simulink model "simulink_controller"  (R2021a)
settings: Solver=FixedStepAuto  StartTime=0.0  StopTime=10.0  RelTol=1e-3
model workspace (MAT data in the model file):
  SL_ROS_VariableLengthArrays_MaxSizes.CommonInfo.ArrayTruncateAction = 'EmitWarning'
  SL_ROS_VariableLengthArrays_MaxSizes.MsgTypeMap = containers.Map
  SL_ROS_VariableLengthArrays_MaxSizes.MsgTypeMap.serialization.keys = {'std_msgs/Float64MultiArray'}
  SL_ROS_VariableLengthArrays_MaxSizes.MsgTypeMap.serialization.values{1}.PropertyName = 'data'
  SL_ROS_VariableLengthArrays_MaxSizes.MsgTypeMap.serialization.values{1}.DataType = 'double'
  SL_ROS_VariableLengthArrays_MaxSizes.MsgTypeMap.serialization.values{1}.MaxLength = 6
  SL_ROS_VariableLengthArrays_MaxSizes.MsgTypeMap.serialization.uniformity = 0
  SL_ROS_VariableLengthArrays_MaxSizes.MsgTypeMap.serialization.keyType = 'char'
  SL_ROS_VariableLengthArrays_MaxSizes.MsgTypeMap.serialization.valueType = 'any'
libraries: ros2lib x3
settings Model: Creator=legacy  LastModifiedBy=legacy
settings OptimizationCC: EnhancedBackFolding=on  PassReuseOutputArgsThreshold=0  ZeroExternalMemoryAtStartup=off  ZeroInternalMemoryAtStartup=off  MaxStackSize=64  OptimizeBlockOrder=speed  DifferentSizesBufferReuse=on  OptimizationCustomize=off
settings DebuggingCC: ParameterTunabilityLossMsg=error
settings HardwareCC: ProdBitPerLong=64  ProdHWDeviceType=Intel->x86-64 (Linux 64)  UseEmbeddedCoderFeatures=off  UseSimulinkCoderFeatures=off
settings SFSimCC: MATLABDynamicMemAlloc=off
settings RTWCC: SystemTargetFile=ert.tlc  HardwareBoard=Robot Operating System 2 (ROS 2)  TemplateMakefile=ert_default_tmf  Toolchain=Colcon Tools  TargetLang=C++
settings CodeAppCC: ForceParamTrailComments=on  OperatorAnnotations=on
settings ERTTargetCC: ERTCustomFileBanners=off  CodeInterfacePackaging=C++ class  SupportContinuousTime=on  SupportNonInlinedSFcns=on  RemoveResetFunc=off  ModelStepFunctionPrototypeControlCompliant=off  RootIOFormat=Structure reference

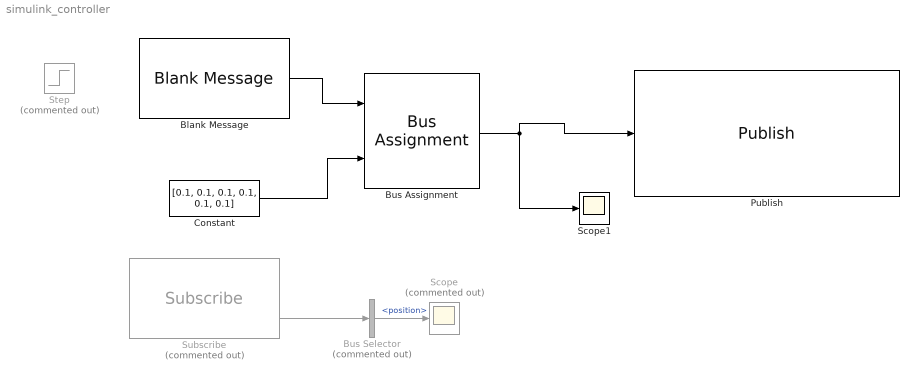
== system simulink_controller ==
  Blank Message : ros2lib/Blank Message  messageType=std_msgs/Float64MultiArray  SampleTime=0.01
      settings: SourceProductBaseCode=RR
  Bus Assignment : BusAssignment  AssignedSignals=data
  Bus Selector : BusSelector  Commented=on  OutputSignals=position
  Constant : Constant  Value=[0.1, 0.1, 0.1, 0.1, 0.1, 0.1]  SampleTime=0.01
  Publish : ros2lib/Publish  topicSource=Select from ROS network  topic=/effort_controllers/commands  messageType=std_msgs/Float64MultiArray  QOSHistory=Keep all  QOSDepth=1  QOSReliability=Best effort  QOSDurability=Volatile
      settings: SourceProductBaseCode=RR
  Scope : Scope  Commented=on
  Scope1 : Scope
  Step : Step  Commented=on  Time=[zeros(1,128)]  Before=[0, 0, 0, 0, 0, 0, zeros(1, 122)]  After=[1, 1, 1, 1, 1, 1, zeros(1, 122)]*10  SampleTime=0.1
  Subscribe : ros2lib/Subscribe  Commented=on  topicSource=Specify your own  topic=/joint_states  messageType=sensor_msgs/JointState  sampleTime=0.01  QOSHistory=Keep last  QOSDepth=1  QOSReliability=Reliable  QOSDurability=Volatile
      settings: SourceProductBaseCode=RR
  wires:
  Blank Message/1 -> Bus Assignment/1
  Bus Assignment/1 -> Publish/1, Scope1/1
  Subscribe/2 -> Bus Selector/1
  Bus Selector/1 -> Scope/1  "<position>"
  Constant/1 -> Bus Assignment/2
